simulink model "Weihnachtsprojekt_Denkinger_Eyes_Schnitzler"  (R2023a)
settings: Solver=VariableStepAuto  StartTime=0.0  StopTime=10.0  RelTol=1e-3
libraries: slpidlib x1
settings Model: Creator=jonat  LastModifiedBy=jonat

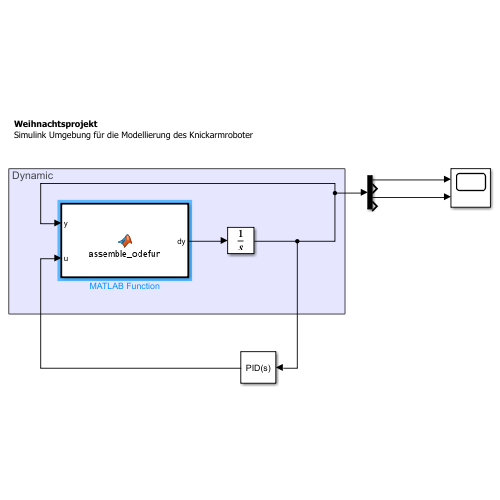
[thumbnail: Simulink's stored preview of the top-level diagram]
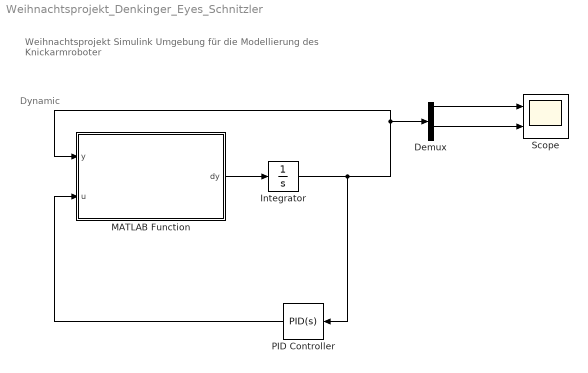
== system Weihnachtsprojekt_Denkinger_Eyes_Schnitzler ==
  note: Dynamic
  note: Weihnachtsprojekt
      | Simulink Umgebung für die Modellierung des Knickarmroboter
  Demux : Demux
  Integrator : Integrator
  MATLAB Function : MATLAB Function  TreatAsAtomicUnit=on
  PID Controller : slpidlib/PID Controller  Controller=PID  Form=Parallel  TimeDomain=Continuous-time  UseExternalTs=off  SampleTime=-1  IntegratorMethod=Forward Euler  FilterMethod=Forward Euler  ControllerParametersSource=internal  P=0  I=0  UseKiTs=off  D=0  N=100  UseFilter=on  TunerSelectOption=Transfer Function Based (PID Tuner App)  InitialConditionSource=internal  InitialConditionForIntegrator=0  InitialConditionForFilter=0  DifferentiatorICPrevScaledInput=0  ExternalReset=none  TrackingMode=off  Kt=1  LimitOutput=off  SatLimitsSource=internal  UpperSaturationLimit=inf  LowerSaturationLimit=-inf  LinearizeAsGain=on  AntiWindupMode=none  Kb=1  LimitIntegrator=off  UpperIntegratorSaturationLimit=inf  LowerIntegratorSaturationLimit=-inf  POutMin=[]  POutMax=[]  IOutMin=[]  IOutMax=[]  DOutMin=[]  DOutMax=[]  NOutMin=[]  NOutMax=[]  SumOutMin=[]  SumOutMax=[]  SaturationOutMin=[]  SaturationOutMax=[]  PParamMin=[]  PParamMax=[]  IParamMin=[]  IParamMax=[]  DParamMin=[]  DParamMax=[]  NParamMin=[]  NParamMax=[]  KbParamMin=[]  KbParamMax=[]  KtParamMin=[]  KtParamMax=[]  KbOutMin=[]  KbOutMax=[]  KtOutMin=[]  KtOutMax=[]  IntegratorOutMin=[]  IntegratorOutMax=[]  FilterOutMin=[]  FilterOutMax=[]  SumI1OutMin=[]  SumI1OutMax=[]  SumI2OutMin=[]  SumI2OutMax=[]  SumI3OutMin=[]  SumI3OutMax=[]  SumI4OutMin=[]  SumI4OutMax=[]  SumDOutMin=[]  SumDOutMax=[]  DifferentiatorOutMin=[]  DifferentiatorOutMax=[]  FilterDiffOutCoefMin=[]  FilterDiffOutCoefMax=[]  ReciprocalOutMin=[]  ReciprocalOutMax=[]  SumDenOutMin=[]  SumDenOutMax=[]  SumNumOutMin=[]  SumNumOutMax=[]  DivideOutMin=[]  DivideOutMax=[]  UdiffTsProdOutMin=[]  UdiffTsProdOutMax=[]  NTsProdOutMin=[]  NTsProdOutMax=[]  UintegralTsProdOutMin=[]  UintegralTsProdOutMax=[]  UngainTsProdOutMin=[]  UngainTsProdOutMax=[]  ClampingZeroOutDataTypeStr=Inherit: Inherit via back propagation  ClampingZeroOutMin=[]  ClampingZeroOutMax=[]  FilterDenConstantOutDataTypeStr=Inherit: Inherit via back propagation  FilterDenConstantOutMin=[]  FilterDenConstantOutMax=[]  PCopyOutDataTypeStr=Inherit: Inherit via back propagation  PCopyOutMin=[]  PCopyOutMax=[]  NCopyOutDataTypeStr=Inherit: Inherit via back propagation  NCopyOutMin=[]  NCopyOutMax=[]  IntegratorContinuousStateAttributes=''  IntegratorStateMustResolveToSignalObject=off  IntegratorRTWStateStorageClass=Auto  FilterContinuousStateAttributes=''  FilterStateMustResolveToSignalObject=off  FilterRTWStateStorageClass=Auto  ParallelPVariant=InternalParameters  IdealPVariant=Disabled  IVariant=InternalParameters  DVariant=InternalParameters  IntegratorVariant=Continuous  SatVariant=Disabled  AWVariant=Passthrough  PCopyVariant=Disabled  TRVariant=Disabled  FdbkBlocksVariant=Forward  IdealPFdbkVariant=Disabled  SatFdbkVariant=Disabled  DerivativeFilterVariant=ContFilter  NVariant=InternalParameters  NCopyVariant=Disabled  FilterICVariant=InternalICsFilter  IntegratorICVariant=InternalICs  ExternalResetVariant=Disabled  TRSumVariant=Passthrough  SumFdbkVariant=Disabled  SumVariant=Sum_PID  TsampFilterVariant=InternalTs  TsampNgainVariant=Passthrough  TsampIntegralVariant=Disabled_SignalSpec  ExternalSaturationOutDataTypeStr=Inherit: Same as second input
  Scope : Scope  NumInputPorts=2
  wires:
  MATLAB Function/1(dy) -> Integrator/1
  Integrator/1 -> PID Controller/1, Demux/1, MATLAB Function/1(y)
  PID Controller/1 -> MATLAB Function/2(u)
  Demux/1 -> Scope/1
  Demux/3 -> Scope/2

== matlab function Weihnachtsprojekt_Denkinger_Eyes_Schnitzler/MATLAB Function ==
  data: y input; dy output; u input
function dy = assemble_odefun(y, u)

dy = zeros(4,1);

alpha = y(1);
alpha_dot = y(2);
beta = y(3);
beta_dot = y(4);
u1 = u(1);
u2 = u(2);
    

%    This function was generated by the Symbolic Math Toolbox version 9.3.
%    07-Jan-2024 10:41:49

t2 = cos(beta);
t3 = sin(alpha);
t4 = sin(beta);
t5 = alpha_dot.^2;
t6 = beta.*2.0;
t7 = beta_dot.^2;
t8 = cos(t6);
t9 = sin(t6);
t10 = alpha+t6;
t15 = beta_dot.*t2.*6.768715453849653e+26;
t17 = t2.*u2.*1.741372640558182e+32;
t11 = sin(t10);
t12 = t8.*4.56261632e+8;
t16 = -t15;
t18 = t5.*t9.*8.416541556157048e+28;
t19 = -t17;
t13 = t12-1.64084533245e+11;
t14 = 1.0./t13;
et1 = alpha_dot.*3.383003808543871e+27-beta_dot.*3.421737133440028e+27-t3.*2.508038558387371e+32+t11.*5.16039204161879e+30+t16+t18+t19+u1.*8.803028385490165e+32;
et2 = u2.*-8.803028385490165e+32+t4.*t5.*8.509500207004381e+29+t4.*t7.*8.509500207004381e+29+alpha_dot.*beta_dot.*t4.*1.701900041400876e+30;
et3 = alpha_dot.*1.691501904271935e+27-beta_dot.*1.378248762589505e+28-t3.*1.254019279193685e+32+t11.*2.580196020809395e+30+t16+t18+t19+u1.*4.401514192745083e+32;
et4 = u2.*-3.54579048775278e+33+sin(alpha+beta).*1.714069110394488e+32-sin(alpha-beta).*1.265840341247194e+31+alpha_dot.*t2.*3.346047528832546e+26+t4.*t5.*3.427559649729151e+30;
et5 = t4.*t7.*4.254750103502191e+29+t7.*t9.*4.208270778078524e+28+t2.*u1.*8.706863202790908e+31+alpha_dot.*beta_dot.*t4.*8.509500207004381e+29+alpha_dot.*beta_dot.*t9.*8.416541556157048e+28;
y_ddot = [t14.*(et1+et2).*(-5.421010862427522e-21);(t14.*(et3+et4+et5))./9.223372036854776e+19];


% Result
dy(1) = y(2);
dy(2) = y_ddot(1);
dy(3) = y(4);
dy(4) = y_ddot(2);
    
end
